simulink model "ex04_host_track_target_demo"  (Simulink 7.3)
settings: Solver=ode45  StartTime=0.0  StopTime=inf  RelTol=1e-3
InitFcn:
  | hsize = 20;
  | sigma = 10;
  | gaus_filt = fspecial('gaussian',hsize , sigma);
undefined symbols (not defined in the file): gray, Low
libraries: vipsnks x7, viptextngfix x2, dspsigattribs x1, waijung_socket_lib x1, dspswit3 x1, vipfilter x1
settings Model: Creator=Krisada  LastModifiedBy=Krisada

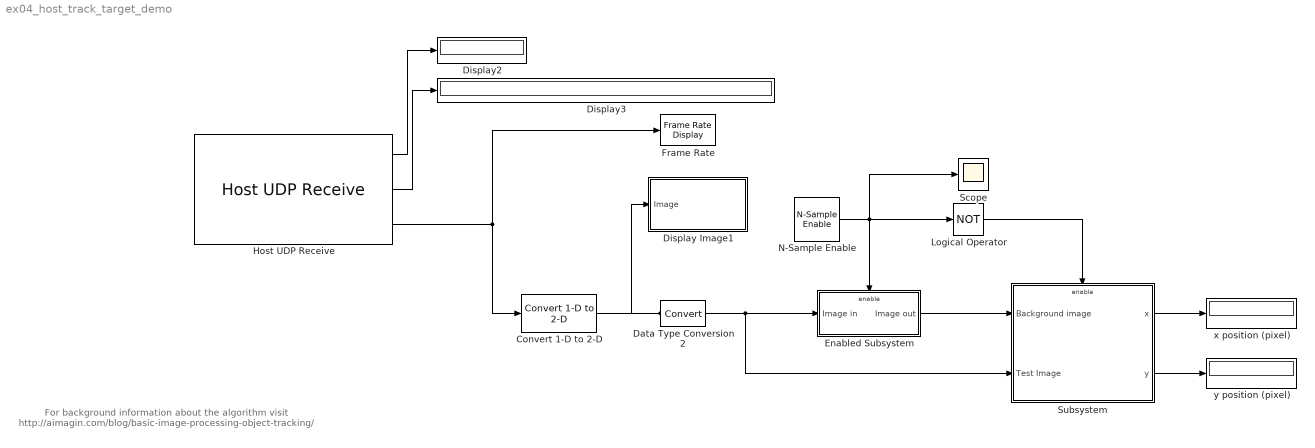
== system ex04_host_track_target_demo ==
  note: For background information about the algorithm visit http://aimagin.com/blog/basic-image-processing-object-tracking/
  Convert 1-D to 2-D : dspsigattribs/Convert 1-D to 2-D  SystemSampleTime=-1  M=160  N=120  frameBasedOut=off
  Data Type Conversion2 : DataTypeConversion  OutDataType=fixdt(1, 16)  OutScaling=2^0
  Display Image1 : Subsystem
  Display2 : Display
  Display3 : Display
  Enabled Subsystem : Subsystem  TreatAsAtomicUnit=on
  Frame Rate : vipsnks/Frame Rate Display  DialogController=vipDDGCreate  DialogControllerArgs=DataTag4  UpdateRate=10
  Host UDP Receive : waijung_socket_lib/Host UDP Receive  conf=HostReceive  protocol=UDP  port=7  address=192.168.1.21  echo=off  transfer=Blocking  timeout=6  datasource=BufferStream  datatype=uint8  datacount=120*160  porttype_double=0  porttype_single=0  porttype_int8=0  porttype_uint8=0  porttype_int16=0  porttype_uint16=0  porttype_int32=0  porttype_uint32=1  portpinstr=0  sampletime=0.1  blockid=HostUDPReceive  inputporttype=[]  inputportwidth=[]  inputportlabel={}  outputporttype=[5,3,3]  outputportwidth=[1,4,19200]  outputportlabel={'Remote Port','Remote IP(1:4)','Data(1:19200)'}  compat=0  optionstring=[]  options=[7,2,1,6000,1]
  Logical Operator : Logic  Operator=NOT  AllPortsSameDT=off  OutDataTypeMode=boolean  LogicDataType=fixdt(0, 8)  OutDataTypeStr=boolean
  N-Sample Enable : dspswit3/N-Sample Enable  N=20  ActiveLevel=Low (0)  reset=off  TriggerType=Rising edge  Ts=-1  DataType=Logical
  Scope : Scope
  Subsystem : Subsystem
  x position (pixel) : Display
  y position (pixel) : Display
  wires:
  Host UDP Receive/3 -> Frame Rate/1, Convert 1-D to 2-D/1
  Host UDP Receive/1 -> Display2/1
  Host UDP Receive/2 -> Display3/1
  N-Sample Enable/1 -> Logical Operator/1, Enabled Subsystem/Enable, Scope/1
  Logical Operator/1 -> Subsystem/Enable
  Data Type Conversion2/1 -> Enabled Subsystem/1(Image in), Subsystem/2(Test Image)
  Subsystem/1(x) -> x position (pixel)/1
  Subsystem/2(y) -> y position (pixel)/1
  Enabled Subsystem/1(Image out) -> Subsystem/1(Background image)
  Convert 1-D to 2-D/1 -> Data Type Conversion2/1, Display Image1/1(Image)

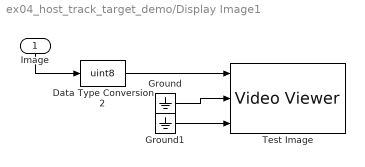
== system ex04_host_track_target_demo/Display Image1 ==
  Image : Inport
  Data Type Conversion2 : DataTypeConversion  OutDataTypeMode=uint8  OutDataType=fixdt(1, 16)  OutScaling=2^0  OutDataTypeStr=uint8
  Ground : Ground
  Ground1 : Ground
  Test Image : vipsnks/Video Viewer  DialogControllerArgs=DataTag1  inputType=Obsolete7b  imagePorts=Separate color signals  useColorMap=off  colormapValue=gray(256)  specRange=off  minInputVal=0  maxInputVal=255  FigPos=[1056 516 410 398]  AxisZoom=on  trueSizedOnce=off  OpenAtMdlStart=on
  wires:
  Image/1 -> Data Type Conversion2/1
  Ground1/1 -> Test Image/3
  Ground/1 -> Test Image/2
  Data Type Conversion2/1 -> Test Image/1

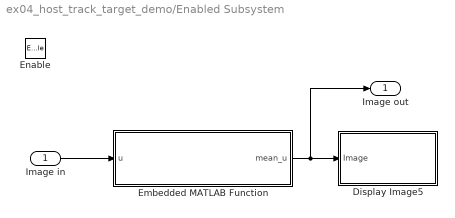
== system ex04_host_track_target_demo/Enabled Subsystem ==
  Image in : Inport  OutDataType=fixdt(1, 16)  OutScaling=2^0
  Enable : EnablePort
  Display Image5 : Subsystem
  Embedded MATLAB Function : Stateflow chart
  Image out : Outport  OutDataType=fixdt(1, 16)  OutScaling=2^0
  wires:
  Embedded MATLAB Function/1(mean_u) -> Display Image5/1(Image), Image out/1
  Image in/1 -> Embedded MATLAB Function/1(u)

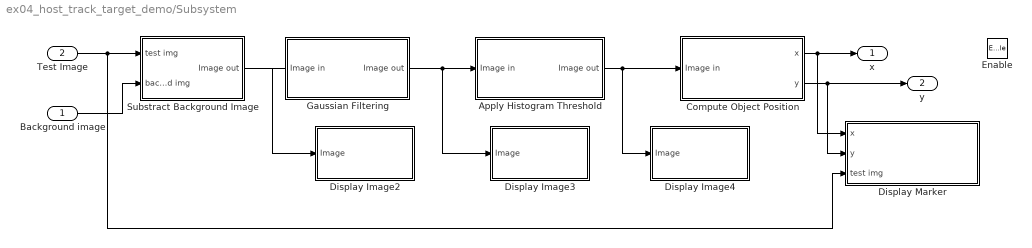
== system ex04_host_track_target_demo/Subsystem ==
  Background image : Inport
  Test Image : Inport  Port=2
  Enable : EnablePort
  Apply Histogram Threshold : Subsystem
  Compute Object Position : Subsystem
  Display Image2 : Subsystem
  Display Image3 : Subsystem
  Display Image4 : Subsystem
  Display Marker : Subsystem
  Gaussian Filtering : Subsystem
  Substract Background Image : Subsystem
  x : Outport
  y : Outport  Port=2
  wires:
  Gaussian Filtering/1(Image out) -> Apply Histogram Threshold/1(Image in), Display Image3/1(Image)
  Substract Background Image/1(Image out) -> Gaussian Filtering/1(Image in), Display Image2/1(Image)
  Apply Histogram Threshold/1(Image out) -> Display Image4/1(Image), Compute Object Position/1(Image in)
  Compute Object Position/1(x) -> Display Marker/1(x), x/1
  Compute Object Position/2(y) -> Display Marker/2(y), y/1
  Test Image/1 -> Substract Background Image/1(test img), Display Marker/3(test img)
  Background image/1 -> Substract Background Image/2(background img)

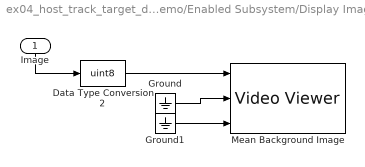
== system ex04_host_track_target_demo/Enabled Subsystem/Display Image5 ==
  Image : Inport
  Data Type Conversion2 : DataTypeConversion  OutDataTypeMode=uint8  OutDataType=fixdt(1, 16)  OutScaling=2^0  OutDataTypeStr=uint8
  Ground : Ground
  Ground1 : Ground
  Mean Background Image : vipsnks/Video Viewer  DialogControllerArgs=DataTag3  inputType=Obsolete7b  imagePorts=Separate color signals  useColorMap=off  colormapValue=gray(256)  specRange=off  minInputVal=0  maxInputVal=255  FigPos=[1498 1035 410 398]  AxisZoom=on  trueSizedOnce=off  OpenAtMdlStart=on
  wires:
  Data Type Conversion2/1 -> Mean Background Image/1
  Ground/1 -> Mean Background Image/2
  Ground1/1 -> Mean Background Image/3
  Image/1 -> Data Type Conversion2/1

== system ex04_host_track_target_demo/Subsystem/Apply Histogram Threshold ==
  Image in : Inport
  Embedded MATLAB Function : Stateflow chart
  Image out : Outport
  wires:
  Image in/1 -> Embedded MATLAB Function/1(img_in)
  Embedded MATLAB Function/1(img_out) -> Image out/1

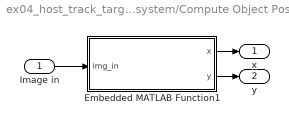
== system ex04_host_track_target_demo/Subsystem/Compute Object Position ==
  Image in : Inport
  Embedded MATLAB Function1 : Stateflow chart
  x : Outport
  y : Outport  Port=2
  wires:
  Image in/1 -> Embedded MATLAB Function1/1(img_in)
  Embedded MATLAB Function1/1(x) -> x/1
  Embedded MATLAB Function1/2(y) -> y/1

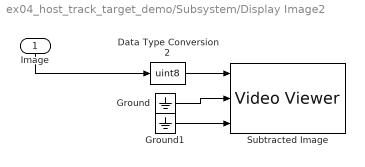
== system ex04_host_track_target_demo/Subsystem/Display Image2 ==
  Image : Inport
  Data Type Conversion2 : DataTypeConversion  OutDataTypeMode=uint8  OutDataType=fixdt(1, 16)  OutScaling=2^0  OutDataTypeStr=uint8
  Ground : Ground
  Ground1 : Ground
  Subtracted Image : vipsnks/Video Viewer  DialogControllerArgs=DataTag6  inputType=Obsolete7b  imagePorts=Separate color signals  useColorMap=off  colormapValue=gray(256)  specRange=off  minInputVal=0  maxInputVal=255  FigPos=[618 1033 410 398]  AxisZoom=on  trueSizedOnce=off  OpenAtMdlStart=on
  wires:
  Data Type Conversion2/1 -> Subtracted Image/1
  Ground/1 -> Subtracted Image/2
  Ground1/1 -> Subtracted Image/3
  Image/1 -> Data Type Conversion2/1

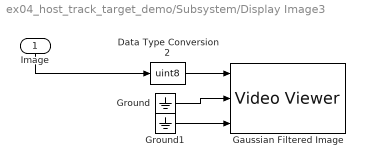
== system ex04_host_track_target_demo/Subsystem/Display Image3 ==
  Image : Inport
  Data Type Conversion2 : DataTypeConversion  OutDataTypeMode=uint8  OutDataType=fixdt(1, 16)  OutScaling=2^0  OutDataTypeStr=uint8
  Gaussian Filtered Image : vipsnks/Video Viewer  DialogControllerArgs=DataTag8  inputType=Obsolete7b  imagePorts=Separate color signals  useColorMap=off  colormapValue=gray(256)  specRange=off  minInputVal=0  maxInputVal=255  FigPos=[622 516 410 398]  AxisZoom=on  trueSizedOnce=off  OpenAtMdlStart=on
  Ground : Ground
  Ground1 : Ground
  wires:
  Data Type Conversion2/1 -> Gaussian Filtered Image/1
  Ground/1 -> Gaussian Filtered Image/2
  Ground1/1 -> Gaussian Filtered Image/3
  Image/1 -> Data Type Conversion2/1

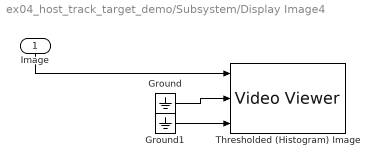
== system ex04_host_track_target_demo/Subsystem/Display Image4 ==
  Image : Inport
  Ground : Ground
  Ground1 : Ground
  Thresholded (Histogram) Image : vipsnks/Video Viewer  DialogControllerArgs=DataTag10  inputType=Obsolete7b  imagePorts=Separate color signals  useColorMap=off  colormapValue=gray(256)  specRange=off  minInputVal=0  maxInputVal=255  FigPos=[1492 513 410 398]  AxisZoom=on  trueSizedOnce=off  OpenAtMdlStart=on
  wires:
  Image/1 -> Thresholded (Histogram) Image/1
  Ground1/1 -> Thresholded (Histogram) Image/3
  Ground/1 -> Thresholded (Histogram) Image/2

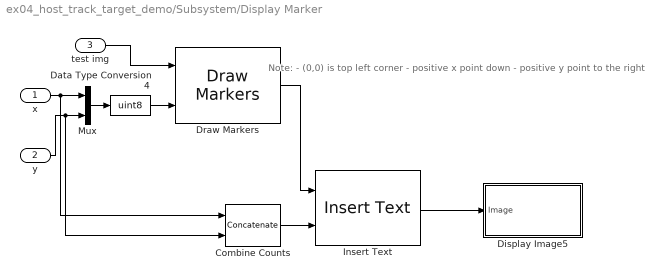
== system ex04_host_track_target_demo/Subsystem/Display Marker ==
  note: Note:
      | - (0,0) is top left corner
      | - positive x point down
      | - positive y point to the right
  x : Inport
  y : Inport  Port=2
  test img : Inport  Port=3
  Combine Counts : Concatenate  Mode=Multidimensional array  ConcatenateDimension=2
  Data Type Conversion4 : DataTypeConversion  OutDataTypeMode=uint8  OutDataType=fixdt(1, 16)  OutScaling=2^0  OutDataTypeStr=uint8
  Display Image5 : Subsystem
  Draw Markers : viptextngfix/Draw Markers  DialogController=vipDDGCreate  DialogControllerArgs=DataTag13  shape=Square  size=5  fill=on  fillClrSource=Specify via dialog  display=White  intensity=200  color=1.5  opacity=0.6  viewport=Entire image  antialiasing=off  inType=Obsolete  imagePorts=One multidimensional signal  prodOutputMode=Binary point scaling  prodOutputWordLength=32  prodOutputFracLength=14  memoryMode=Specify word length  memoryWordLength=16  memoryFracLength=14  roundingMode=Floor  overflowMode=off
  Insert Text : viptextngfix/Insert Text  DialogController=vipDDGCreate  DialogControllerArgs=DataTag14  inputType=Obsolete  theText='x: %3.2f, y: %3.2f'  fontFace=LucidaSansRegular  dummyVar1=0  blockFontSize=12  antiAliased=on  getTextLocFrom=Specify via dialog  textLoc=[20 150]  getTextColorFrom=Specify via dialog  textColor=[0 0 0]  getTextIntensityFrom=Specify via dialog  textIntensity=0  getTextOpacityFrom=Specify via dialog  textOpacity=1.0  dummyVar2=0  dummyVar3=0  dummyVar4=0  imagePorts=One multidimensional signal  isInputTransposed=off
  Mux : Mux  Inputs=2
  wires:
  Mux/1 -> Data Type Conversion4/1
  Data Type Conversion4/1 -> Draw Markers/2
  test img/1 -> Draw Markers/1
  x/1 -> Mux/1, Combine Counts/1
  y/1 -> Mux/2, Combine Counts/2
  Draw Markers/1 -> Insert Text/1
  Combine Counts/1 -> Insert Text/2
  Insert Text/1 -> Display Image5/1(Image)

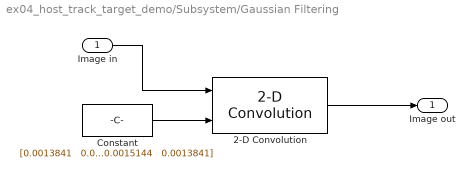
== system ex04_host_track_target_demo/Subsystem/Gaussian Filtering ==
  Image in : Inport
  2-D Convolution : vipfilter/2-D Convolution  DialogController=vipDDGCreate  DialogControllerArgs=DataTag15  outSize=Same as input port I1  normalize=off  outputMode=Binary point scaling  outputWordLength=32  outputFracLength=12  prodOutputMode=Binary point scaling  prodOutputWordLength=32  prodOutputFracLength=10  roundingMode=Floor  overflowMode=off
  Constant : Constant  Value=|  VectorParams1D=off  OutDataType=fixdt(1, 16)  OutScaling=2^0
      | [0.0013841   0.0015144   0.0016406   0.0017595   0.0018683   0.0019641   0.0020443   0.0021065   0.0021491   0.0021707   0.0021707   0.0021491   0.0021065   0.0020443   0.0019641   0.0018683   0.0017595   0.0016406   0.0015144   0.0013841
      | 0.0015144   0.0016571   0.0017951   0.0019252   0.0020443   0.0021491   0.0022368   0.0023049   0.0023515   0.0023751   0.0023751   0.0023515   0.0023049   0.0022368   0.0021491   0.0020443   0.0019252   0.0017951   0.0016571   0.0015144
      | 0.0016406   0.0017951   0.0019446   0.0020856   0.0022145   0.0023281   0.0024231   0.0024969   0.0025473   0.0025729   0.0025729   0.0025473   0.0024969   0.0024231   0.0023281   0.0022145   0.0020856   0.0019446   0.0017951   0.0016406
      | 0.0017595   0.0019252   0.0020856   0.0022368   0.0023751   0.0024969   0.0025988   0.0026779    0.002732   0.0027595   0.0027595    0.002732   0.0026779   0.0025988   0.0024969   0.0023751   0.0022368   0.0020856   0.0019252   0.0017595
      | 0.0018683   0.0020443   0.0022145   0.0023751    0.002522   0.0026513   0.0027595   0.0028435    0.002901   0.0029301   0.0029301    0.002901   0.0028435   0.0027595   0.0026513    0.002522   0.0023751   0.0022145   0.0020443   0.0018683
      | 0.0019641   0.0021491   0.0023281   0.0024969   0.0026513   0.0027872    0.002901   0.0029893   0.0030497   0.0030804   0.0030804   0.0030497   0.0029893    0.002901   0.0027872   0.0026513   0.0024969   0.0023281   0.0021491   0.0019641
      | 0.0020443   0.0022368   0.0024231   0.0025988   0.0027595    0.002901   0.0030194   0.0031113   0.0031742   0.0032061   0.0032061   0.0031742   0.0031113   0.0030194    0.002901   0.0027595   0.0025988   0.0024231   0.0022368   0.0020443
      | 0.0021065   0.0023049   0.0024969   0.0026779   0.0028435   0.0029893   0.0031113   0.0032061   0.0032708   0.0033037   0.0033037   0.0032708   0.0032061   0.0031113   0.0029893   0.0028435   0.0026779   0.0024969   0.0023049   0.0021065
      | 0.0021491   0.0023515   0.0025473    0.002732    0.002901   0.0030497   0.0031742   0.0032708   0.0033369   0.0033705   0.0033705   0.0033369   0.0032708   0.0031742   0.0030497    0.002901    0.002732   0.0025473   0.0023515   0.0021491
      | 0.0021707   0.0023751   0.0025729   0.0027595   0.0029301   0.0030804   0.0032061   0.0033037   0.0033705   0.0034043   0.0034043   0.0033705   0.0033037   0.0032061   0.0030804   0.0029301   0.0027595   0.0025729   0.0023751   0.0021707
      | 0.0021707   0.0023751   0.0025729   0.0027595   0.0029301   0.0030804   0.0032061   0.0033037   0.0033705   0.0034043   0.0034043   0.0033705   0.0033037   0.0032061   0.0030804   0.0029301   0.0027595   0.0025729   0.0023751   0.0021707
      | 0.0021491   0.0023515   0.0025473    0.002732    0.002901   0.0030497   0.0031742   0.0032708   0.0033369   0.0033705   0.0033705   0.0033369   0.0032708   0.0031742   0.0030497    0.002901    0.002732   0.0025473   0.0023515   0.0021491
      | 0.0021065   0.0023049   0.0024969   0.0026779   0.0028435   0.0029893   0.0031113   0.0032061   0.0032708   0.0033037   0.0033037   0.0032708   0.0032061   0.0031113   0.0029893   0.0028435   0.0026779   0.0024969   0.0023049   0.0021065
      | 0.0020443   0.0022368   0.0024231   0.0025988   0.0027595    0.002901   0.0030194   0.0031113   0.0031742   0.0032061   0.0032061   0.0031742   0.0031113   0.0030194    0.002901   0.0027595   0.0025988   0.0024231   0.0022368   0.0020443
      | 0.0019641   0.0021491   0.0023281   0.0024969   0.0026513   0.0027872    0.002901   0.0029893   0.0030497   0.0030804   0.0030804   0.0030497   0.0029893    0.002901   0.0027872   0.0026513   0.0024969   0.0023281   0.0021491   0.0019641
      | 0.0018683   0.0020443   0.0022145   0.0023751    0.002522   0.0026513   0.0027595   0.0028435    0.002901   0.0029301   0.0029301    0.002901   0.0028435   0.0027595   0.0026513    0.002522   0.0023751   0.0022145   0.0020443   0.0018683
      | 0.0017595   0.0019252   0.0020856   0.0022368   0.0023751   0.0024969   0.0025988   0.0026779    0.002732   0.0027595   0.0027595    0.002732   0.0026779   0.0025988   0.0024969   0.0023751   0.0022368   0.0020856   0.0019252   0.0017595
      | 0.0016406   0.0017951   0.0019446   0.0020856   0.0022145   0.0023281   0.0024231   0.0024969   0.0025473   0.0025729   0.0025729   0.0025473   0.0024969   0.0024231   0.0023281   0.0022145   0.0020856   0.0019446   0.0017951   0.0016406
      | 0.0015144   0.0016571   0.0017951   0.0019252   0.0020443   0.0021491   0.0022368   0.0023049   0.0023515   0.0023751   0.0023751   0.0023515   0.0023049   0.0022368   0.0021491   0.0020443   0.0019252   0.0017951   0.0016571   0.0015144
      | 0.0013841   0.0015144   0.0016406   0.0017595   0.0018683   0.0019641   0.0020443   0.0021065   0.0021491   0.0021707   0.0021707   0.0021491   0.0021065   0.0020443   0.0019641   0.0018683   0.0017595   0.0016406   0.0015144   0.0013841]
  Image out : Outport
  wires:
  Constant/1 -> 2-D Convolution/2
  Image in/1 -> 2-D Convolution/1
  2-D Convolution/1 -> Image out/1

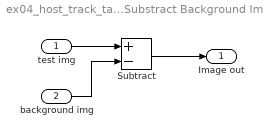
== system ex04_host_track_target_demo/Subsystem/Substract Background Image ==
  test img : Inport
  background img : Inport  Port=2
  Subtract : Sum  Inputs=+-  OutDataType=fixdt(1, 16)  OutScaling=2^-10  RndMeth=Nearest
  Image out : Outport
  wires:
  test img/1 -> Subtract/1
  Subtract/1 -> Image out/1
  background img/1 -> Subtract/2

== system ex04_host_track_target_demo/Subsystem/Display Marker/Display Image5 ==
  Image : Inport
  Data Type Conversion2 : DataTypeConversion  OutDataTypeMode=uint8  OutDataType=fixdt(1, 16)  OutScaling=2^0  OutDataTypeStr=uint8
  Traked Object : vipsnks/Video Viewer  DialogControllerArgs=DataTag12  inputType=Obsolete7b  imagePorts=Separate color signals  useColorMap=off  colormapValue=gray(256)  specRange=off  minInputVal=0  maxInputVal=255  FigPos=[1056 1035 410 398]  AxisZoom=on  trueSizedOnce=off  OpenAtMdlStart=on
  wires:
  Data Type Conversion2/1 -> Traked Object/1, Traked Object/2, Traked Object/3
  Image/1 -> Data Type Conversion2/1

== matlab function Subsystem/Compute Object Position/Embedded MATLAB Function1 ==
  data: img_in input double; x output double; y output double
function [x,y] = fcn(img_in)
	%#eml
	
	% size 352, 288
	sumx = 0;
	sumx_cnt = 0;
    for j = 1:120
		for i = 1:160
			if (img_in(i,j) ~= 0)
				sumx = sumx + i;
				sumx_cnt = sumx_cnt + 1;
			end
		end
	end
	if (sumx ~= 0)
		x = sumx/sumx_cnt;
	else
		x = 100;
	end
	
	sumy = 0;
	sumy_cnt = 0;
	for i = 1:160
		for j = 1:120
			if (img_in(i,j) ~= 0)
				sumy = sumy + j;
				sumy_cnt = sumy_cnt + 1;
			end
		end
	end
	if (sumy ~= 0)
		y = sumy/sumy_cnt;
	else
		y = 100;
	end

== matlab function Subsystem/Apply Histogram Threshold/Embedded MATLAB Function ==
  data: img_in input double; img_out output double
function img_out = fcn(img_in)
	%#eml
	
	img_out = (img_in < -20);

== matlab function Enabled Subsystem/Embedded MATLAB Function ==
  data: u input double; mean_u output double
function mean_u = recursive_mean(u)
    %#eml
    
    persistent ubar
    persistent cnt
    
    if isempty(ubar)
        ubar = zeros(size(u));
        cnt = 0;
    end
    cnt = cnt + 1;
    
    ubar = (((cnt-1)/cnt)*ubar) + ((1/cnt)*u);
    mean_u = ubar;
